simulink model "ESSOneYearInOneMinute_R2015a"  (R2020b)
settings: Solver=ode23tb  StartTime=0  StopTime=365*24*60*60  RelTol=1e-4  EnableMultiTasking=on
StartFcn:
  | tic
StopFcn:
  | toc
values from neighbouring files (symbols this model uses):
  BP1 = [1:24]'    [Build_LoadProfile_Datasets.m]    (also in LoadProfile_Datasets.mat = [1 2 3 4 5 6 7 8 9 10 11 12 ... (24 elements, 24x1)])
  BP2 = [1:3]    [Build_LoadProfile_Datasets.m]    (also in LoadProfile_Datasets.mat = [1 2 3])
  BP3 = [1:2]    [Build_LoadProfile_Datasets.m]    (also in LoadProfile_Datasets.mat = [1 2])
  LoadProfile_Data = [1 2 3 4 5 6 7 8 9 10 11 12 ... (144 elements, 24x3x2)]    [LoadProfile_Datasets.mat]
undefined symbols (not defined in the file or in its folder): A, B, C, D1, Dd, Delta, j, StationData
libraries: powerlib x43, simulink x10, powerlib_meascontrol x8
(part 1 of 2)
settings Model: SimulationMode=accelerator  Creator=at4494  LastModifiedBy=Jared Gooding
settings DataIOCC: LimitDataPoints=on  SaveFormat=Array  SignalLoggingSaveFormat=ModelDataLogs  SaveOutput=off  SaveTime=off  ReturnWorkspaceOutputs=off
settings OptimizationCC: LifeSpan=inf
settings DebuggingCC: UnderspecifiedInitializationDetection=Classic  MergeDetectMultiDrivingBlocksExec=none  SolverPrmCheckMsg=warning  MultiTaskDSMMsg=warning  MultiTaskCondExecSysMsg=none  SFUnexpectedBacktrackingDiag=warning  SFNoUnconditionalDefaultTransitionDiag=warning  SFExecutionAtInitializationDiag=none  ArithmeticOperatorsInVariantConditions=warning
settings HardwareCC: ProdBitPerPointer=32  ProdBitPerSizeT=32  ProdBitPerPtrDiffT=32  ProdLargestAtomicFloat=None  ProdIntDivRoundTo=Undefined  ProdEndianess=Unspecified  ProdWordSize=32  ProdHWDeviceType=32-bit Generic
settings ModelReferenceCC: PropagateSignalLabelsOutOfModel=off
settings SFSimCC: SimUseLocalCustomCode=off  CustomCodeUndefinedFunction=UseInterfaceOnly
settings RTWCC: RTWUseLocalCustomCode=off
settings CodeAppCC: StateflowObjectComments=on
settings GRTTargetCC: TargetLangStandard=C89/C90 (ANSI)
settings ConfigComp: CovMetricSettings=dw  CovSaveCumulativeToWorkspaceVar=on  CovSaveSingleToWorkspaceVar=on  CovExternalEMLEnable=off  CovSFcnEnable=off
settings SimscapeCC: SimscapeNormalizeSystem=off

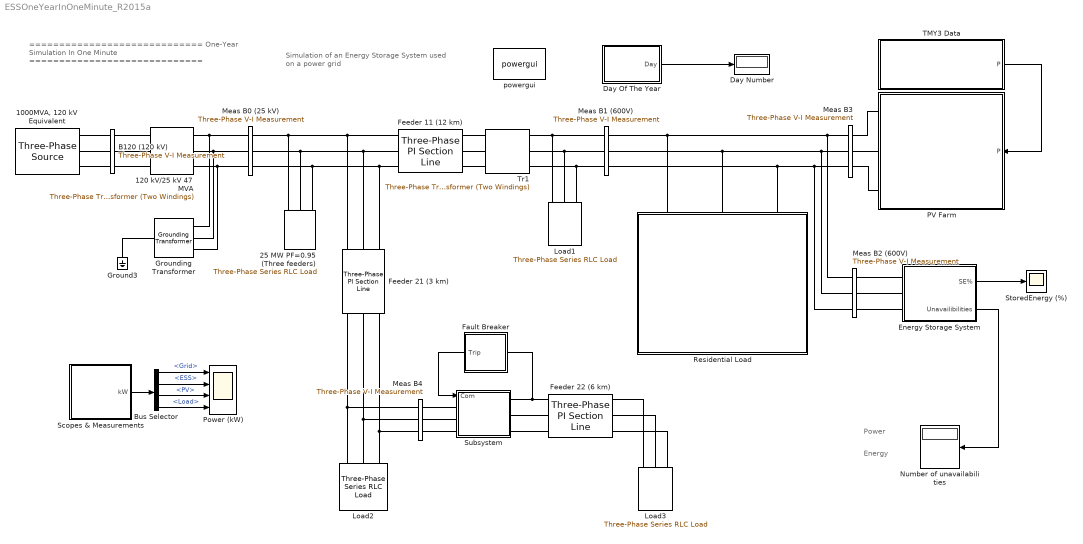
== system ESSOneYearInOneMinute_R2015a ==
  note: Simulation of an Energy Storage
      | System used on a power grid
  note: Power
  note: =============================
      | One-Year Simulation In One Minute
      | =============================
  note: Energy
  " Feeder 11 (12 km)" : powerlib/Elements/Three-Phase PI Section Line  LConnTagsString=a|b|c  RConnTagsString=A|B|C  Length=12  Frequency=60  Resistances=[ 0.104 0.357]  Inductances="[1.048e-3  3.483e-3]"  Capacitances="[ 11.212e-09   4.8118e-09]"
  " Feeder 21 (3 km)" : powerlib/Elements/Three-Phase PI Section Line  LConnTagsString=a|b|c  RConnTagsString=A|B|C  Length=3  Frequency=60  Resistances=[ 0.104 0.357]  Inductances="[1.048e-3  3.483e-3]"  Capacitances="[ 11.212e-09   4.8118e-09]"
  "1000MVA, 120 kV Equivalent" : powerlib/Electrical Sources/Three-Phase Source  InternalConnection=Yg  VoltagePhases=off  Voltage=120e3*1.07  PhaseAngle=0  Voltage_phases=[25e3 25e3 25e3]/sqrt(3)  PhaseAngles_phases=[0 -120 +120]  Frequency=60  NonIdealSource=on  SpecifyImpedance=on  Resistance=0.8929  Inductance=16.58e-3  ShortCircuitLevel=1000e6  BaseVoltage=120e3  XRratio=7  BusType=swing  Pref=0  Qref=0  Prefabc=[10e3, 10e3, 10e3]  Qrefabc=[0, 0, 0]  Qmin=-inf  Qmax=inf
  120 kV/25 kV 47 MVA : powerlib/Elements/Three-Phase Transformer (Two Windings)  Winding1Connection=Yg  Winding2Connection=Delta (D1)  CoreType=Three single-phase transformers  SetSaturation=off  Hysteresis=off  DataFile='basic_model'  SetInitialFlux=off  Measurements=None  UNITS=pu  NominalPower=[47e6 60]  Winding1="[ 120e3  0.185/2/25   0.185/2 ]"  Winding2="[ 25e3  0.185/2/25  0.185/2]"  Rm=500  Lm=500  L0=0.5  Saturation="[ 0,0  ;  0.005,1.2  ;  1.0,1.4 ]"  InitialFluxes=[ 0.8 , -0.8 , 0.7 ]  BreakLoop=off  DiscreteSolver=Trapezoidal iterative  DataType=off  TransfoNumber=0
  25 MW PF=0.95 (Three feeders) : powerlib/Elements/Three-Phase Series RLC Load  LConnTagsString=A|B|C  Configuration=Y (grounded)  NominalVoltage=25e3  Vabc=[1e3 1e3 1e3]  Vabcp=[1e3 1e3 1e3]  NominalFrequency=60  UnbalancedPower=off  ActivePower=25e6  InductivePower=25e6*sqrt(1/0.95^2 - 1)  CapacitivePower=0  Pabc=[10e3 9e3 11e3]  QLabc=[100 90 110]  QCabc=[100 90 110]  Pabcp=[10e3 9e3 11e3]  QLabcp=[100 90 110]  QCabcp=[100 90 110]  Measurements=None  LoadType=constant Z
  B120 (120 kV) : powerlib/Measurements/Three-Phase V-I Measurement  VoltageMeasurement=no  SetLabelV=on  LabelV=Vabc_B120_1  Vpu=on  VpuLL=off  CurrentMeasurement=no  SetLabelI=on  LabelI=Iabc_B120  Ipu=off  Pbase=100e6  Vbase=120e3  OutputType=Complex  PhasorSimulation=on  PSBequivalent=0
  Bus Selector : BusSelector  OutputSignals=Grid,ESS,PV,Load
  Day Number : Display
  Day Of The Year : Subsystem
      mask Display: image(imread('Calendar.ico'))
  Energy Storage System : Subsystem  mask(Generic Energy Storage System){Pnom=275, kWh_Rated=1000, Initial_kWh_pc=90, Efficiency=96, Pmax_Grid=1000, Ki=1000, MinMax=[ 10  90 ], ChargingPower=150}
      mask prompts: Pnom "Rated power in kW"; kWh_Rated "Rated capacity in kWh"; Initial_kWh_pc "Initial stored energy in % of rated capacity"; Efficiency "System efficiency in %"; Pmax_Grid "Maximum power allowed from the grid (kW)"; Ki "Regulator integral gain:"; MinMax "Range of operation [ min  max ] in % of Stored Energy"; ChargingPower "Maximum charging power (kW) during night time:"
      mask help:
      | Model a generic Energy Storage System (ESS) connected to grid through an inverter. The storage technology can be Battery, Flywheel, SuperCapacitor, ...
      |
      | Look Under Mask to see how the model is built.
      mask init:
      | Min=MinMax(1);
      | Max=MinMax(2);
      | Plimit=Pnom*1e3;
      mask DialogControl Container4 Prompt: Power
      mask DialogControl Container7 Prompt: Control
      mask Display: image(imread('Energy.jpg'))
  Fault Breaker : Subsystem  mask(Single-phase Fault Breaker){Day=50, Hour=9, Minute=28, Second=9, FaultDuration=0.2, Ron=0.1}
      mask prompts: FaultDuration "Fault duration (s):"; Ron "Fault resistance (ohm):"
      mask init:
      | T1=(Day-1)*24*60*60;  % Day in seconds
      | T2=(Hour-1)*60*60;    % Hour in seconds
      | T3=(Minute-1)*60;  % Minute in seconds
      | Ton=T1+T2+T3+(Second-1);    % Beginning of fault (s)
      | Toff=Ton+FaultDuration; % End of fault (s)
      mask TypeOptions Day: 1 |      2 |      3 |      4 |      5 |      6 |      7 |      8 |      9 |     10 |     11 |     12 |     13 |     14 |     15 |     16 |     17 |     18 |     19 |     20 |     21 |     22 |     23 |     24 |     25 |     26 |     27 |     28 |     29 |     30 |     31 |     32 |     33 |     34 |     35 |     36 |     37 |     38 |     39 |     40 |     41 |     42 |     43 |     44 |     45 |     46 |     47 |     48 |     49 |     50 |     51 |     52 |     53 |     54 |     55 |     56 |     57 |     58 |     59 |     60 |     61 |     62 |     63 |     64 |     65 |     66 |     67 |     68 |     69 |     70 |     71 |     72 |     73 |     74 |     75 |     76 |     77 |     78 |     79 |     80 |     81 |     82 |     83 |     84 |     85 |     86 |     87 |     88 |     89 |     90 |     91 |     92 |     93 |     94 |     95 |     96 |     97 |     98 |     99 |    100 |    101 |    102 |    103 |    104 |    105 |    106 |    107 |    108 |    109 |    110 |    111 |    112 |    113 |    114 |    115 |    116 |    117 |    118 |    119 |    120 |    121 |    122 |    123 |    124 |    125 |    126 |    127 |    128 |    129 |    130 |    131 |    132 |    133 |    134 |    135 |    136 |    137 |    138 |    139 |    140 |    141 |    142 |    143 |    144 |    145 |    146 |    147 |    148 |    149 |    150 |    151 |    152 |    153 |    154 |    155 |    156 |    157 |    158 |    159 |    160 |    161 |    162 |    163 |    164 |    165 |    166 |    167 |    168 |    169 |    170 |    171 |    172 |    173 |    174 |    175 |    176 |    177 |    178 |    179 |    180 |    181 |    182 |    183 |    184 |    185 |    186 |    187 |    188 |    189 |    190 |    191 |    192 |    193 |    194 |    195 |    196 |    197 |    198 |    199 |    200 |    201 |    202 |    203 |    204 |    205 |    206 |    207 |    208 |    209 |    210 |    211 |    212 |    213 |    214 |    215 |    216 |    217 |    218 |    219 |    220 |    221 |    222 |    223 |    224 |    225 |    226 |    227 |    228 |    229 |    230 |    231 |    232 |    233 |    234 |    235 |    236 |    237 |    238 |    239 |    240 |    241 |    242 |    243 |    244 |    245 |    246 |    247 |    248 |    249 |    250 |    251 |    252 |    253 |    254 |    255 |    256 |    257 |    258 |    259 |    260 |    261 |    262 |    263 |    264 |    265 |    266 |    267 |    268 |    269 |    270 |    271 |    272 |    273 |    274 |    275 |    276 |    277 |    278 |    279 |    280 |    281 |    282 |    283 |    284 |    285 |    286 |    287 |    288 |    289 |    290 |    291 |    292 |    293 |    294 |    295 |    296 |    297 |    298 |    299 |    300 |    301 |    302 |    303 |    304 |    305 |    306 |    307 |    308 |    309 |    310 |    311 |    312 |    313 |    314 |    315 |    316 |    317 |    318 |    319 |    320 |    321 |    322 |    323 |    324 |    325 |    326 |    327 |    328 |    329 |    330 |    331 |    332 |    333 |    334 |    335 |    336 |    337 |    338 |    339 |    340 |    341 |    342 |    343 |    344 |    345 |    346 |    347 |    348 |    349 |    350 |    351 |    352 |    353 |    354 |    355 |    356 |    357 |    358 |    359 |    360 |    361 |    362 |    363 |    364 |    365
      mask TypeOptions Hour: 0 |      1 |      2 |      3 |      4 |      5 |      6 |      7 |      8 |      9 |     10 |     11 |     12 |     13 |     14 |     15 |     16 |     17 |     18 |     19 |     20 |     21 |     22 |     23
      mask TypeOptions Minute: 0 |      1 |      2 |      3 |      4 |      5 |      6 |      7 |      8 |      9 |     10 |     11 |     12 |     13 |     14 |     15 |     16 |     17 |     18 |     19 |     20 |     21 |     22 |     23 |     24 |     25 |     26 |     27 |     28 |     29 |     30 |     31 |     32 |     33 |     34 |     35 |     36 |     37 |     38 |     39 |     40 |     41 |     42 |     43 |     44 |     45 |     46 |     47 |     48 |     49 |     50 |     51 |     52 |     53 |     54 |     55 |     56 |     57 |     58 |     59
      mask TypeOptions Second: 0 |      1 |      2 |      3 |      4 |      5 |      6 |      7 |      8 |      9 |     10 |     11 |     12 |     13 |     14 |     15 |     16 |     17 |     18 |     19 |     20 |     21 |     22 |     23 |     24 |     25 |     26 |     27 |     28 |     29 |     30 |     31 |     32 |     33 |     34 |     35 |     36 |     37 |     38 |     39 |     40 |     41 |     42 |     43 |     44 |     45 |     46 |     47 |     48 |     49 |     50 |     51 |     52 |     53 |     54 |     55 |     56 |     57 |     58 |     59
      mask DialogControl Control2 Prompt: Fault timing:
  Feeder 22 (6 km) : powerlib/Elements/Three-Phase PI Section Line  LConnTagsString=a|b|c  RConnTagsString=A|B|C  Length=6  Frequency=60  Resistances=[ 0.104 0.357]  Inductances="[1.048e-3  3.483e-3]"  Capacitances="[ 11.212e-09   4.8118e-09]"
  Ground3 : powerlib/Elements/Ground  LConnTagsString=a
  "Grounding Transformer " : powerlib/Elements/Grounding Transformer   UNITS=pu  NominalPower="[10e6   60]"  NominalVoltage=25e3  ZeroSequenceImpedance_pu=[0.25 7.5]/(25e3^2/10e6)  MagnetizationBranch_pu=[500 500]  ZeroSequenceImpedance_SI=[0.052083 589.05]  MagnetizationBranch_SI=[1041.7 3.927e+005]  Measurements=None
      settings: SourceProductBaseCode=PS
  Load1 : powerlib/Elements/Three-Phase Series RLC Load  LConnTagsString=A|B|C  Configuration=Y (grounded)  NominalVoltage=600  Vabc=[1e3 1e3 1e3]  Vabcp=[1e3 1e3 1e3]  NominalFrequency=60  UnbalancedPower=off  ActivePower=50e3  InductivePower=0  CapacitivePower=0  Pabc=[10e3 9e3 11e3]  QLabc=[100 90 110]  QCabc=[100 90 110]  Pabcp=[10e3 9e3 11e3]  QLabcp=[100 90 110]  QCabcp=[100 90 110]  Measurements=None  LoadType=constant Z
  Load2 : powerlib/Elements/Three-Phase Series RLC Load  LConnTagsString=A|B|C  Configuration=Y (grounded)  NominalVoltage=25e3  Vabc=[1e3 1e3 1e3]  Vabcp=[1e3 1e3 1e3]  NominalFrequency=60  UnbalancedPower=off  ActivePower=2e6  InductivePower=0.4e6  CapacitivePower=0  Pabc=[10e3 9e3 11e3]  QLabc=[100 90 110]  QCabc=[100 90 110]  Pabcp=[10e3 9e3 11e3]  QLabcp=[100 90 110]  QCabcp=[100 90 110]  Measurements=None  LoadType=constant Z
  Load3 : powerlib/Elements/Three-Phase Series RLC Load  LConnTagsString=A|B|C  Configuration=Y (grounded)  NominalVoltage=25e3  Vabc=[1e3 1e3 1e3]  Vabcp=[1e3 1e3 1e3]  NominalFrequency=60  UnbalancedPower=off  ActivePower=5e6  InductivePower=0.6e6  CapacitivePower=0  Pabc=[10e3 9e3 11e3]  QLabc=[100 90 110]  QCabc=[100 90 110]  Pabcp=[10e3 9e3 11e3]  QLabcp=[100 90 110]  QCabcp=[100 90 110]  Measurements=None  LoadType=constant Z
  "Meas B0 (25 kV) " : powerlib/Measurements/Three-Phase V-I Measurement  VoltageMeasurement=phase-to-ground  SetLabelV=on  LabelV=Vabc_B0  Vpu=off  VpuLL=off  CurrentMeasurement=yes  SetLabelI=on  LabelI=Iabc_B0  Ipu=off  Pbase=10e6  Vbase=25e3  OutputType=Complex  PhasorSimulation=on  PSBequivalent=0
  Meas B1 (600V) : powerlib/Measurements/Three-Phase V-I Measurement  VoltageMeasurement=phase-to-ground  SetLabelV=on  LabelV=Vabc_B1  Vpu=off  VpuLL=off  CurrentMeasurement=yes  SetLabelI=on  LabelI=Iabc_B1  Ipu=off  Pbase=100e6  Vbase=500e3  OutputType=Complex  PhasorSimulation=on  PSBequivalent=0
  Meas B2 (600V) : powerlib/Measurements/Three-Phase V-I Measurement  VoltageMeasurement=phase-to-ground  SetLabelV=on  LabelV=Vabc_B2  Vpu=off  VpuLL=off  CurrentMeasurement=yes  SetLabelI=on  LabelI=Iabc_B2  Ipu=off  Pbase=100e6  Vbase=500e3  OutputType=Complex  PhasorSimulation=on  PSBequivalent=0
  Meas B3 : powerlib/Measurements/Three-Phase V-I Measurement  VoltageMeasurement=phase-to-ground  SetLabelV=on  LabelV=Vabc_B3  Vpu=off  VpuLL=off  CurrentMeasurement=yes  SetLabelI=on  LabelI=Iabc_B3  Ipu=off  Pbase=100e6  Vbase=500e3  OutputType=Complex  PhasorSimulation=on  PSBequivalent=0
  Meas B4 : powerlib/Measurements/Three-Phase V-I Measurement  VoltageMeasurement=phase-to-ground  SetLabelV=on  LabelV=Vabc_B4  Vpu=off  VpuLL=off  CurrentMeasurement=yes  SetLabelI=on  LabelI=Iabc_B4  Ipu=off  Pbase=100e6  Vbase=500e3  OutputType=Complex  PhasorSimulation=on  PSBequivalent=0
  Number of unavailabilities : Display
  PV Farm : Subsystem
      mask Display: image(imread('PV_Farm.jpg'))
  Power (kW) : Scope  NumInputPorts=4
  Residential Load : Subsystem  mask(Dynamic Load based on Load Profiles){DatasetsNumber=Southwest USA, Vnom=600, Pnom_Load=1500, PF=0.95, np_nq=[ 1.8  1.4 ], PlotData_On=off}
      mask prompts: Vnom "Nominal L-L voltage (Vrms)"; Pnom_Load "Nominal load (kVA)"; PF "Power factor ( 0 to 1)"; np_nq "Parameters [ np  nq ]"; PlotData_On "Plot load profile"
      mask help:
      | Implements a three-phase, three-wire dynamic load based on Load Profiles.
      | Active power P and reactive power Q absorbed by the load vary as function of positive-sequence voltage V and load profiles data.
      | The profiles are daily load profiles specified on an hourly basis. For each load profile, the user specifies summer and winter data.
      | P & Q vary as follows:
      | P=P_LoadProfile*(V/Vo)^np
      | Q=Q_LoadProfile*(V/Vo)^nq
      | Note: If np=nq=2, the load behaves as constant impedance load.
      | See documentation below to define additionnal load profiles.
      mask init:
      | BlockName=gcb;
      | load LoadProfile_Datasets
      | np=np_nq(1);
      | nq=np_nq(2);
      | if PlotData_On==1
      |     clf
      |     plot([1:24],LoadProfile_Data(:,2,DatasetsNumber),'r')
      |     hold on
      |     plot([1:24],LoadProfile_Data(:,3,DatasetsNumber),'b')
      |     grid
      |     if DatasetsNumber==1
      |         str='Southwest, USA';
      |     else
      |         str='Northeast, USA';
      |     end
      |     title(['Load profile:',  str ])
      |     ylabel('% of nominal load')
      |     xlabel('Hour of the day')
      |     axis([0 24 0 100])
      |     legend('Summer', 'Winter', 'Location','NorthWest')
      |     set_param(BlockName,'PlotData_On', 'off')
      | end
      settings: AttributesFormatString=Profile:%<DatasetsNumber>
      mask TypeOptions DatasetsNumber: Southwest USA | Northeast USA
      mask DialogControl Control3 Prompt: Documentation
      mask DialogControl Control3 Callback: open('Build_LoadProfile_Datasets.m')
      mask DialogControl Control2 Prompt: Load Profile:
      mask Display: image(imread('Residential.jpg'))
  Scopes & Measurements : Subsystem
  StoredEnergy (%) : Scope
  Subsystem : Subsystem
      mask Display: disp('Three-phase\nBreaker')
  TMY3 Data : Subsystem  mask(TMY3 -to- Power){SortByState=on, ListNum_State=Binghamton Edwin A Link Field, NY, ListNum_Name=Rock Springs Arpt [Green River - UO], WY, IrradianceType=Global Horizontal Irradiance (Wh/m2), TotalArea=3000, Efficiency=20, PlotData_On=off}
      mask prompts: SortByState "Sort site name by state:"; TotalArea "Solar panels total area (m2):"; Efficiency "Overall system efficiency (%):"; PlotData_On "Plot meteorological data"
      mask help:
      | Convert TMY3 solar irradiance data to Power.
      |
      | TMY3 are data files for the typical meteorological year (TMY) data sets
      | derived from the 1961-1990 and 1991-2005 National Solar Radiation
      | Data Base (NSRDB) archives. The files contain hourly values of solar radiation and meteorological elements for a 1-year period.
      |
      | TMY3 files have been produced by NREL's Electric Systems Center under
      | the Solar Resource Characterization Project, which is funded and
      | monitored by the U.S. Department of Energy's Energy Efficiency and
      | Renewable Energy Office.
      |
      | Look Under Mask for additionnal information
      mask init:
      | BlockName=gcb;
      | % Mask parameters visibility:
      | %
      | MV = get_param(BlockName,'MaskVisibilities');
      | MV{3}='off';
      | if SortByState==1
      | 	MV{2}='on';
      |     MV{3}='off';
      |     str_NameState=ListNum_State;
      | else
      |     MV{2}='off';
      |     MV{3}='on';
      |     str_NameState=ListNum_Name;
      | end
      | set_param(BlockName,'MaskVisibilities',MV)
      | %
      | load StationData_NEW
      | max=size(StationData,2);
      | for i=1:max
      |     if strcmp([StationData(i).Name{1}, ', ', StationData(i).State{1}],str_NameState)
      |        Index=StationData(i).NumberByState;
      |     end
      | end
      | if IrradianceType==1
      |     IrradianceTable=StationData(Index).GHIWm2;
      | else
      |     IrradianceTable=StationData(Index).DNIWm2;
      | end
      | if PlotData_On==1
      |     h2=figure;
      |     set(h2,'Name',[StationData(Index).Name{1}, ', ', StationData(Index).State{1}]);
      |     ScreenS=get(0,'Screensize');
      |     set(h2,'Position',[ScreenS(3)/14 ScreenS(4)/12 ScreenS(3)/2.4 ScreenS(4)/1.25])
      |     subplot(3,1,1)
      |     plot([1:size(StationData(Index).GHIWm2,1)]',StationData(Index).GHIWm2)
      |     title('Global Horizontal Irradiance')
      |     ylabel('Wh/m2')
      |     grid
      |     subplot(3,1,2)
      |     plot([1:size(StationData(Index).DHIWm2,1)]',StationData(Index).DHIWm2)
      |     title('Diffuse Horizontal Irradiance')
      |     ylabel('Wh/m2')
      |     grid
      |     subplot(3,1,3)
      |     plot([1:size(StationData(Index).DNIWm2,1)]',StationData(Index).DNIWm2)
      |     title('Direct Normal Irradiance')
      |     ylabel('Wh/m2')
      |     xlabel('Time of the Year in Hours')
      |     %
      |     h3=figure;
      |     set(h3,'Name',[StationData(Index).Name{1}, ', ', StationData(Index).State{1}]);
      |     ScreenS=get(0,'Screensize');
      |     set(h3,'Position',[ScreenS(3)/2 ScreenS(4)/12 ScreenS(3)/2.4 ScreenS(4)/1.25])
      |     subplot(2,1,1)
      |     plot([1:size(StationData(Index).Temperature,1)]',StationData(Index).Temperature)
      |     title('Temperature')
      |     ylabel('C')
      |     grid
      |     subplot(2,1,2)
      |     plot([1:size(StationData(Index).WindSpeed,1)]',StationData(Index).WindSpeed)
      |     title('Wind Speed')
      |     ylabel('m/s')
      |     grid
      |     xlabel('Time of the Year in Hours')
      |     set_param(BlockName,'PlotData_On', 'off')
      | end
      mask TypeOptions ListNum_State: Birmingham Municipal AP, AL | Huntsville Intl/Jones Field, AL | Mobile Regional AP, AL | Montgomery Dannelly Field, AL | Fort Smith Regional AP, AR | Little Rock Adams Field, AR | Phoenix Sky Harbor Intl AP, AZ | Prescott Love Field, AZ | Tucson International AP, AZ | Arcata Airport, CA | Bakersfield Meadows Field, CA | Bishop Airport, CA | Daggett Barstow-Daggett AP, CA | Fresno Yosemite Intl AP, CA | Long Beach Daugherty Fld, CA | Los Angeles Intl Arpt, CA | Redding Municipal Arpt, CA | Sacramento Executive Arpt, CA | San Diego Lindbergh Field, CA | San Francisco Intl AP, CA | Santa Barbara Municipal AP, CA | Santa Maria Public Arpt, CA | Stockton Metropolitan Arpt, CA | Alamosa San Luis Valley Rgnl, CO | Colorado Springs Muni AP, CO | Denver Intl AP, CO | Grand Junction Walker Field, CO | Limon, CO | Pueblo Memorial AP, CO | Bridgeport Sikorsky Memorial, CT | Hartford Bradley Intl AP, CT | Wilmington New Castle Cnty AP, DE | Daytona Beach Intl AP, FL | Fort Myers Page Field, FL | Gainesville Regional AP, FL | Jacksonville Intl Arpt, FL | Key West Intl Arpt, FL | Miami Intl AP, FL | Orlando Intl Arpt, FL | Pensacola Regional AP, FL | Tallahassee Regional AP [ISIS], FL | Tampa International AP, FL | Vero Beach Municipal Arpt, FL | West Palm Beach Intl Arpt, FL | Athens Ben Epps AP, GA | Atlanta Hartsfield Intl AP, GA | Augusta Bush Field, GA | Columbus Metropolitan Arpt, GA | Macon Middle Ga Regional AP, GA | Savannah Intl AP, GA | Hilo International AP, HI | Honolulu Intl Arpt, HI | Kahului Airport, HI | Lihue Airport, HI | Boise Air Terminal [UO], ID | Lewiston Nez Perce Cnty AP, ID | Pocatello Regional AP, ID | Chicago Ohare Intl AP, IL | Moline Quad City Intl AP, IL | Peoria Greater Peoria AP, IL | Rockford Greater Rockford AP, IL | Springfield Capital AP, IL | Evansville Regional AP, IN | Fort Wayne Intl AP, IN | Indianapolis Intl AP, IN | South Bend Michiana Rgnl AP, IN | Des Moines Intl AP, IA | Dubuque Regional AP, IA | Mason City Municipal Arpt, IA | Sioux City Sioux Gateway AP, IA | Waterloo Municipal AP, IA | Concordia Blosser Muni AP, KS | Dodge City Regional AP, KS | Goodland Renner Field, KS | Russell Municipal AP, KS | Topeka Municipal AP, KS | Wichita Mid-Continent AP, KS | Cincinnati Northern Ky AP, KY | Jackson Julian Carroll AP, KY | Lexington Bluegrass AP, KY | Louisville Standiford Field, KY | Paducah Barkley Regional AP, KY | Baton Rouge Ryan Arpt, LA | Lake Charles Regional Arpt, LA | New Orleans Intl Arpt, LA | Shreveport Regional Arpt, LA | Bangor International AP, ME | Caribou Municipal Arpt, ME | Portland Intl Jetport, ME | Baltimore Blt-Washngtn Int'l, MD | Boston Logan Int'l Arpt, MA | Worchester Regional Arpt, MA | Alpena County Regional AP, MI | Detroit City Airport, MI | Detroit Metropolitan Arpt, MI | Flint Bishop Intl Arpt, MI | Grand Rapids Kent County Int', MI | Houghton Lake Roscommon Co Ar, MI | Lansing Capital City Arpt, MI | Muskegon County Arpt, MI | Sault Ste Marie Sanderson Fie, MI | Traverse City Cherry Capital, MI | Duluth International Arpt, MN | International Falls Intl AP, MN | Minneapolis-St Paul Int'l Arp, MN | Rochester International Arpt, MN | St Cloud Regional Arpt, MN | Jackson International AP, MS | Meridian Key Field, MS | Tupelo C D Lemons Arpt, MS | Columbia Regional Airport, MO | Kansas City Int'l Arpt, MO | Springfield Regional Arpt, MO | St Louis Lambert Int'l Arpt, MO | St Louis Spirit of St Louis Airport, MO | Billings Logan Int'l Arpt, MT | Glasgow Intl Arpt, MT | Great Falls Intl Arpt, MT | Havre City-County AP, MT | Helena Regional Airport, MT | Kalispell Glacier Pk Int'l Ar, MT | Missoula International AP, MT | Grand Island Central NE Regio, NE | Lincoln Municipal Arpt, NE | Norfolk Karl Stefan Mem Arpt, NE | North Platte Regional AP, NE | Omaha Eppley Airfield, NE | Scottsbluff W B Heilig Field, NE | Valentine Miller Field, NE | Ely Yelland Field, NV | Las Vegas McCarran Intl AP, NV | Lovelock Derby Field, NV | Mercury Desert Rock AP [SURFRAD], NV | Reno Tahoe International AP, NV | Tonopah Airport, NV | Winnemucca Municipal Arpt, NV | Concord Municipal Arpt, NH | Atlantic City Intl AP, NJ | Newark International Arpt, NJ | Albuquerque Intl Arpt [ISIS], NM | Gallup Sen Clarke Fld, NM | Roswell Industrial Air Park, NM | Albany County AP, NY | Binghamton Edwin A Link Field, NY | Buffalo Niagara Intl AP, NY | Islip Long Isl MacArthur AP, NY | Massena AP, NY | New York J F Kennedy Int'l Ar, NY | New York Laguardia Arpt, NY | Rochester Greater Rochester I, NY | Syracuse Hancock Int'l Arpt, NY | Asheville Regional Arpt, NC | Charlotte Douglas Intl Arpt, NC | Greensboro Piedmont Triad Int, NC | Raleigh Durham International, NC | Wilmington International Arpt, NC | Bismarck Municipal Arpt [ISIS], ND | Fargo Hector International AP, ND | Minot FAA AP, ND | Williston Sloulin Intl AP, ND | Akron Akron-Canton Reg AP, OH | Cleveland Hopkins Intl AP, OH | Columbus Port Columbus Intl A, OH | Dayton International Airport, OH | Mansfield Lahm Municipal Arpt, OH | Toledo Express Airport, OH | Youngstown Regional Airport, OH | Oklahoma City Will Rogers Wor, OK | Tulsa International Airport, OK | Astoria Regional Airport, OR | Burns Municipal Arpt [UO], OR | Eugene Mahlon Sweet Arpt [UO], OR | Medford Rogue Valley Intl AP [Ashland - UO], OR | Pendleton E Or Regional AP, OR | Salem McNary Field, OR | Allentown Lehigh Valley Intl, PA | Bradford Regional AP, PA | Erie International AP, PA | Middletown Harrisburg Intl AP, PA | Philadelphia International AP, PA | Pittsburgh International AP, PA | Wilkes-Barre Scranton Intl AP, PA | Williamsport Regional AP, PA | Providence T F Green State Ar, RI | Charleston Intl Arpt, SC | Columbia Metro Arpt, SC | Greer Greenv'l-Spartanbrg AP, SC | Aberdeen Regional Arpt, SD | Huron Regional Arpt, SD | Pierre Municipal AP, SD | Rapid City Regional Arpt, SD | Sioux Falls Foss Field, SD | Bristol Tri City Airport, TN | Chattanooga Lovell Field AP, TN | Knoxville McGhee Tyson AP, TN | Memphis International AP, TN | Nashville International AP, TN | Abilene Regional AP [UT], TX | Amarillo International AP [Canyon - UT], TX | Austin Mueller Municipal AP [UT], TX | Brownsville S Padre Isl Intl, TX | Corpus Christi Intl Arpt [UT], TX | Dallas-Fort Worth Intl AP, TX | El Paso International AP [UT], TX | Houston Bush Intercontinental, TX | Lubbock International AP, TX | Lufkin Angelina Co, TX | Midland International AP, TX | Port Arthur Jefferson County, TX | San Angelo Mathis Field, TX | San Antonio Intl AP, TX | Victoria Regional AP, TX | Waco Regional AP, TX | Cedar City Municipal AP, UT | Salt Lake City Int'l Arpt [ISIS], UT | Burlington International AP, VT | Lynchburg Regional Arpt, VA | Norfolk International AP, VA | Richmond International AP, VA | Roanoke Regional AP, VA | Washington DC Dulles Int'l Ar [Sterling - ISIS], VA | Washington DC Reagan AP, VA | Olympia Airport, WA | Quillayute State Airport, WA | Seattle Seattle-Tacoma Intl A, WA | Spokane International AP [Cheney - UO], WA | Stampede Pass, WA | Yakima Air Terminal, WA | Beckley Raleigh Co Mem AP, WV | Charleston Yeager Arpt, WV | Elkins Elkins-Randolph Co Arp, WV | Huntington Tri-State Arpt, WV | Eau Claire County AP, WI | Green Bay Austin Straubel Int, WI | La Crosse Municipal Arpt, WI | Madison Dane Co Regional Arpt [ISIS], WI | Milwaukee Mitchell Intl AP, WI | Casper Natrona Co Intl AP, WY | Cheyenne Municipal Arpt, WY | Lander Hunt Field, WY | Rock Springs Arpt [Green River - UO], WY | Sheridan County Arpt, WY
      mask TypeOptions ListNum_Name: Aberdeen Regional Arpt, SD | Abilene Regional AP [UT], TX | Akron Akron-Canton Reg AP, OH | Alamosa San Luis Valley Rgnl, CO | Albany County AP, NY | Albuquerque Intl Arpt [ISIS], NM | Allentown Lehigh Valley Intl, PA | Alpena County Regional AP, MI | Amarillo International AP [Canyon - UT], TX | Arcata Airport, CA | Asheville Regional Arpt, NC | Astoria Regional Airport, OR | Athens Ben Epps AP, GA | Atlanta Hartsfield Intl AP, GA | Atlantic City Intl AP, NJ | Augusta Bush Field, GA | Austin Mueller Municipal AP [UT], TX | Bakersfield Meadows Field, CA | Baltimore Blt-Washngtn Int'l, MD | Bangor International AP, ME | Baton Rouge Ryan Arpt, LA | Beckley Raleigh Co Mem AP, WV | Billings Logan Int'l Arpt, MT | Binghamton Edwin A Link Field, NY | Birmingham Municipal AP, AL | Bishop Airport, CA | Bismarck Municipal Arpt [ISIS], ND | Boise Air Terminal [UO], ID | Boston Logan Int'l Arpt, MA | Bradford Regional AP, PA | Bridgeport Sikorsky Memorial, CT | Bristol Tri City Airport, TN | Brownsville S Padre Isl Intl, TX | Buffalo Niagara Intl AP, NY | Burlington International AP, VT | Burns Municipal Arpt [UO], OR | Caribou Municipal Arpt, ME | Casper Natrona Co Intl AP, WY | Cedar City Municipal AP, UT | Charleston Intl Arpt, SC | Charleston Yeager Arpt, WV | Charlotte Douglas Intl Arpt, NC | Chattanooga Lovell Field AP, TN | Cheyenne Municipal Arpt, WY | Chicago Ohare Intl AP, IL | Cincinnati Northern Ky AP, KY | Cleveland Hopkins Intl AP, OH | Colorado Springs Muni AP, CO | Columbia Metro Arpt, SC | Columbia Regional Airport, MO | Columbus Metropolitan Arpt, GA | Columbus Port Columbus Intl A, OH | Concord Municipal Arpt, NH | Concordia Blosser Muni AP, KS | Corpus Christi Intl Arpt [UT], TX | Daggett Barstow-Daggett AP, CA | Dallas-Fort Worth Intl AP, TX | Dayton International Airport, OH | Daytona Beach Intl AP, FL | Denver Intl AP, CO | Des Moines Intl AP, IA | Detroit City Airport, MI | Detroit Metropolitan Arpt, MI | Dodge City Regional AP, KS | Dubuque Regional AP, IA | Duluth International Arpt, MN | Eau Claire County AP, WI | El Paso International AP [UT], TX | Elkins Elkins-Randolph Co Arp, WV | Ely Yelland Field, NV | Erie International AP, PA | Eugene Mahlon Sweet Arpt [UO], OR | Evansville Regional AP, IN | Fargo Hector International AP, ND | Flint Bishop Intl Arpt, MI | Fort Myers Page Field, FL | Fort Smith Regional AP, AR | Fort Wayne Intl AP, IN | Fresno Yosemite Intl AP, CA | Gainesville Regional AP, FL | Gallup Sen Clarke Fld, NM | Glasgow Intl Arpt, MT | Goodland Renner Field, KS | Grand Island Central NE Regio, NE | Grand Junction Walker Field, CO | Grand Rapids Kent County Int', MI | Great Falls Intl Arpt, MT | Green Bay Austin Straubel Int, WI | Greensboro Piedmont Triad Int, NC | Greer Greenv'l-Spartanbrg AP, SC | Hartford Bradley Intl AP, CT | Havre City-County AP, MT | Helena Regional Airport, MT | Hilo International AP, HI | Honolulu Intl Arpt, HI | Houghton Lake Roscommon Co Ar, MI | Houston Bush Intercontinental, TX | Huntington Tri-State Arpt, WV | Huntsville Intl/Jones Field, AL | Huron Regional Arpt, SD | Indianapolis Intl AP, IN | International Falls Intl AP, MN | Islip Long Isl MacArthur AP, NY | Jackson International AP, MS | Jackson Julian Carroll AP, KY | Jacksonville Intl Arpt, FL | Kahului Airport, HI | Kalispell Glacier Pk Int'l Ar, MT | Kansas City Int'l Arpt, MO | Key West Intl Arpt, FL | Knoxville McGhee Tyson AP, TN | La Crosse Municipal Arpt, WI | Lake Charles Regional Arpt, LA | Lander Hunt Field, WY | Lansing Capital City Arpt, MI | Las Vegas McCarran Intl AP, NV | Lewiston Nez Perce Cnty AP, ID | Lexington Bluegrass AP, KY | Lihue Airport, HI | Limon, CO | Lincoln Municipal Arpt, NE | Little Rock Adams Field, AR | Long Beach Daugherty Fld, CA | Los Angeles Intl Arpt, CA | Louisville Standiford Field, KY | Lovelock Derby Field, NV | Lubbock International AP, TX | Lufkin Angelina Co, TX | Lynchburg Regional Arpt, VA | Macon Middle Ga Regional AP, GA | Madison Dane Co Regional Arpt [ISIS], WI | Mansfield Lahm Municipal Arpt, OH | Mason City Municipal Arpt, IA | Massena AP, NY | Medford Rogue Valley Intl AP [Ashland - UO], OR | Memphis International AP, TN | Mercury Desert Rock AP [SURFRAD], NV | Meridian Key Field, MS | Miami Intl AP, FL | Middletown Harrisburg Intl AP, PA | Midland International AP, TX | Milwaukee Mitchell Intl AP, WI | Minneapolis-St Paul Int'l Arp, MN | Minot FAA AP, ND | Missoula International AP, MT | Mobile Regional AP, AL | Moline Quad City Intl AP, IL | Montgomery Dannelly Field, AL | Muskegon County Arpt, MI | Nashville International AP, TN | New Orleans Intl Arpt, LA | New York J F Kennedy Int'l Ar, NY | New York Laguardia Arpt, NY | Newark International Arpt, NJ | Norfolk International AP, VA | Norfolk Karl Stefan Mem Arpt, NE | North Platte Regional AP, NE | Oklahoma City Will Rogers Wor, OK | Olympia Airport, WA | Omaha Eppley Airfield, NE | Orlando Intl Arpt, FL | Paducah Barkley Regional AP, KY | Pendleton E Or Regional AP, OR | Pensacola Regional AP, FL | Peoria Greater Peoria AP, IL | Philadelphia International AP, PA | Phoenix Sky Harbor Intl AP, AZ | Pierre Municipal AP, SD | Pittsburgh International AP, PA | Pocatello Regional AP, ID | Port Arthur Jefferson County, TX | Portland Intl Jetport, ME | Prescott Love Field, AZ | Providence T F Green State Ar, RI | Pueblo Memorial AP, CO | Quillayute State Airport, WA | Raleigh Durham International, NC | Rapid City Regional Arpt, SD | Redding Municipal Arpt, CA | Reno Tahoe International AP, NV | Richmond International AP, VA | Roanoke Regional AP, VA | Rochester Greater Rochester I, NY | Rochester International Arpt, MN | Rock Springs Arpt [Green River - UO], WY | Rockford Greater Rockford AP, IL | Roswell Industrial Air Park, NM | Russell Municipal AP, KS | Sacramento Executive Arpt, CA | Salem McNary Field, OR | Salt Lake City Int'l Arpt [ISIS], UT | San Angelo Mathis Field, TX | San Antonio Intl AP, TX | San Diego Lindbergh Field, CA | San Francisco Intl AP, CA | Santa Barbara Municipal AP, CA | Santa Maria Public Arpt, CA | Sault Ste Marie Sanderson Fie, MI | Savannah Intl AP, GA | Scottsbluff W B Heilig Field, NE | Seattle Seattle-Tacoma Intl A, WA | Sheridan County Arpt, WY | Shreveport Regional Arpt, LA | Sioux City Sioux Gateway AP, IA | Sioux Falls Foss Field, SD | South Bend Michiana Rgnl AP, IN | Spokane International AP [Cheney - UO], WA | Springfield Capital AP, IL | Springfield Regional Arpt, MO | St Cloud Regional Arpt, MN | St Louis Lambert Int'l Arpt, MO | St Louis Spirit of St Louis Airport, MO | Stampede Pass, WA | Stockton Metropolitan Arpt, CA | Syracuse Hancock Int'l Arpt, NY | Tallahassee Regional AP [ISIS], FL | Tampa International AP, FL | Toledo Express Airport, OH | Tonopah Airport, NV | Topeka Municipal AP, KS | Traverse City Cherry Capital, MI | Tucson International AP, AZ | Tulsa International Airport, OK | Tupelo C D Lemons Arpt, MS | Valentine Miller Field, NE | Vero Beach Municipal Arpt, FL | Victoria Regional AP, TX | Waco Regional AP, TX | Washington DC Dulles Int'l Ar [Sterling - ISIS], VA | Washington DC Reagan AP, VA | Waterloo Municipal AP, IA | West Palm Beach Intl Arpt, FL | Wichita Mid-Continent AP, KS | Wilkes-Barre Scranton Intl AP, PA | Williamsport Regional AP, PA | Williston Sloulin Intl AP, ND | Wilmington International Arpt, NC | Wilmington New Castle Cnty AP, DE | Winnemucca Municipal Arpt, NV | Worchester Regional Arpt, MA | Yakima Air Terminal, WA | Youngstown Regional Airport, OH
      mask TypeOptions IrradianceType: Global Horizontal Irradiance (Wh/m2) | Direct Normal Irradiance (Wh/m2)
      mask DialogControl Control2 Prompt: Site name:
      mask DialogControl Control3 Prompt: Choose irradiance type:
      mask Display: disp([StationData(Index).Name{1},', ',StationData(Index).State{1}])
  Tr1 : powerlib/Elements/Three-Phase Transformer (Two Windings)  Winding1Connection=Yg  Winding2Connection=Yg  CoreType=Three single-phase transformers  SetSaturation=off  Hysteresis=off  DataFile='basic_model'  SetInitialFlux=off  Measurements=None  UNITS=pu  NominalPower=[10e6 60]  Winding1=[ 25e3 0.05/30/2 0.01 ]  Winding2=[ 600 0.05/30/2 0.04 ]  Rm=200  Lm=200  L0=0.5  Saturation="[ 0,0  ;  0.005,1.2  ;  1.0,1.4 ]"  InitialFluxes=[ 0.8 , -0.8 , 0.7 ]  BreakLoop=off  DiscreteSolver=Trapezoidal iterative  DataType=off  TransfoNumber=1
  powergui : powerlib/powergui  Priority=1  SimulationMode=Phasor  SampleTime=50e-6  frequency=60  Iterations=50  frequencyindice=60  Pbase=100e6  ErrMax=1e-4  UnitsV=kV  UnitsW=MW  buscounter=0  FunctionMessages=off  echomessages=off  EnableUseOfTLC=off  CurrentSourceSwitches=off  DisableSnubberDevices=off  DisableRonSwitches=off  DisableVfSwitches=off  DisplayEquations=off  AutomaticDiscreteSolvers=off  SolverType=Tustin  Interpol=off  ExternalGateDelay=off  methode=off  Ts=0  x0status=blocks  SPID=off  SwTol=0  HookPort=off  NonlinearTolerance=1e-4  nMaxIteration=100  ContinueOnMaxIteration=off  RestoreLinks=warning  ResistiveCurrentMeasurement=off  Frange=[0:2:500]  Ylog=off  Xlog=on  ShowGrid=off  save=off  variable=ZData  structure=0  ZoomFFT=off  StartTime=0.0  cycles=1  DisplayStyle=1  fundamental=60  FreqAxis=off  MaxFrequency=1000  frequencyindicesteady=1  RmsSteady=1  display=off
  wires:
  Day Of The Year/1(Day) -> Day Number/1
  Scopes & Measurements/1(kW) -> Bus Selector/1
  Bus Selector/3 -> Power (kW)/3  "<PV>"
  Bus Selector/2 -> Power (kW)/2  "<ESS>"
  Bus Selector/1 -> Power (kW)/1  "<Grid>"
  Bus Selector/4 -> Power (kW)/4  "<Load>"
  TMY3 Data/1(P) -> PV Farm/1(P)
  Energy Storage System/1(SE%) -> StoredEnergy (%)/1
  Fault Breaker/1(Trip) -> Subsystem/1(Com)
  Energy Storage System/2(Unavailibilities) -> Number of unavailabilities/1
  connections:
  Tr1/RConn1 -- Meas B1 (600V)/LConn1 -- Load1/LConn1
  Tr1/RConn2 -- Load1/LConn2 -- Meas B1 (600V)/LConn2
  Tr1/RConn3 -- Load1/LConn3 -- Meas B1 (600V)/LConn3
  " Feeder 11 (12 km)"/RConn1 -- Tr1/LConn1
  " Feeder 11 (12 km)"/RConn2 -- Tr1/LConn2
  " Feeder 11 (12 km)"/RConn3 -- Tr1/LConn3
  "Meas B0 (25 kV) "/RConn1 -- " Feeder 11 (12 km)"/LConn1 -- " Feeder 21 (3 km)"/LConn1 -- 25 MW PF=0.95 (Three feeders)/LConn1
  "Meas B0 (25 kV) "/RConn2 -- " Feeder 21 (3 km)"/LConn2 -- " Feeder 11 (12 km)"/LConn2 -- 25 MW PF=0.95 (Three feeders)/LConn2
  " Feeder 11 (12 km)"/LConn3 -- "Meas B0 (25 kV) "/RConn3 -- 25 MW PF=0.95 (Three feeders)/LConn3 -- " Feeder 21 (3 km)"/LConn3
  Meas B3/RConn1 -- Meas B1 (600V)/RConn1 -- Residential Load/LConn1 -- Meas B2 (600V)/RConn1
  Meas B2 (600V)/RConn3 -- Meas B1 (600V)/RConn3 -- Residential Load/LConn3 -- Meas B3/RConn3
  Meas B2 (600V)/RConn2 -- Meas B1 (600V)/RConn2 -- Residential Load/LConn2 -- Meas B3/RConn2
  Load2/LConn3 -- " Feeder 21 (3 km)"/RConn3 -- Meas B4/LConn3
  " Feeder 21 (3 km)"/RConn1 -- Load2/LConn1 -- Meas B4/LConn1
  " Feeder 21 (3 km)"/RConn2 -- Meas B4/LConn2 -- Load2/LConn2
  Feeder 22 (6 km)/RConn1 -- Load3/LConn1
  Feeder 22 (6 km)/RConn2 -- Load3/LConn2
  Feeder 22 (6 km)/RConn3 -- Load3/LConn3
  120 kV/25 kV 47 MVA/RConn3 -- "Meas B0 (25 kV) "/LConn3 -- "Grounding Transformer "/LConn3
  "Meas B0 (25 kV) "/LConn1 -- "Grounding Transformer "/LConn1 -- 120 kV/25 kV 47 MVA/RConn1
  120 kV/25 kV 47 MVA/RConn2 -- "Meas B0 (25 kV) "/LConn2 -- "Grounding Transformer "/LConn2
  Ground3/LConn1 -- "Grounding Transformer "/RConn1
  "1000MVA, 120 kV Equivalent"/RConn3 -- B120 (120 kV)/LConn3
  120 kV/25 kV 47 MVA/LConn1 -- B120 (120 kV)/RConn1
  120 kV/25 kV 47 MVA/LConn3 -- B120 (120 kV)/RConn3
  120 kV/25 kV 47 MVA/LConn2 -- B120 (120 kV)/RConn2
  "1000MVA, 120 kV Equivalent"/RConn2 -- B120 (120 kV)/LConn2
  "1000MVA, 120 kV Equivalent"/RConn1 -- B120 (120 kV)/LConn1
  PV Farm/RConn1 -- Meas B3/LConn1
  PV Farm/RConn2 -- Meas B3/LConn2
  PV Farm/RConn3 -- Meas B3/LConn3
  Meas B4/RConn1 -- Subsystem/LConn1
  Meas B4/RConn2 -- Subsystem/LConn2
  Meas B4/RConn3 -- Subsystem/LConn3
  Subsystem/RConn1 -- Fault Breaker/LConn1 -- Feeder 22 (6 km)/LConn1
  Subsystem/RConn2 -- Feeder 22 (6 km)/LConn2
  Subsystem/RConn3 -- Feeder 22 (6 km)/LConn3
  Meas B2 (600V)/LConn1 -- Energy Storage System/LConn1
  Meas B2 (600V)/LConn2 -- Energy Storage System/LConn2
  Energy Storage System/LConn3 -- Meas B2 (600V)/LConn3

== system ESSOneYearInOneMinute_R2015a/Day Of The Year ==
  Add : Sum
  Compare To Zero : simulink/Logic and Bit Operations/Compare To Zero  relop===  OutDataTypeStr=boolean
  Constant : Constant
  Counter : Subsystem
  Hour -to- Day : Gain  Gain=1/24
  Rounding Function : Rounding  Operator=fix
  Sawtooth Generator : powerlib_meascontrol/Pulse & Signal Generators/Sawtooth Generator  Freq=1/60/60  Phase=180  Ts=0
  Day : Outport
  wires:
  Sawtooth Generator/1 -> Add/1
  Compare To Zero/1 -> Counter/Enable
  Add/1 -> Compare To Zero/1
  Constant/1 -> Add/2
  Counter/1(Out1) -> Hour -to- Day/1
  Hour -to- Day/1 -> Rounding Function/1
  Rounding Function/1 -> Day/1

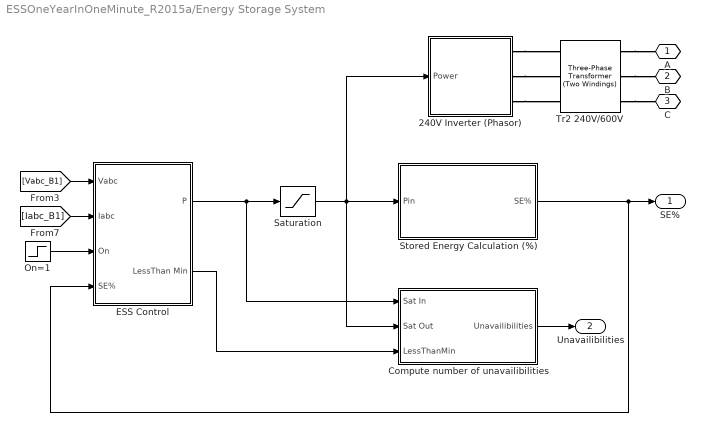
== system ESSOneYearInOneMinute_R2015a/Energy Storage System ==
  240V Inverter (Phasor) : Subsystem
  Compute number of unavailibilities : Subsystem
  ESS Control : Subsystem
  On=1 : Step  Time=0.01*24*60*60  Before=1  SampleTime=0
  Saturation : Saturate  UpperLimit=Pnom*1e3  LowerLimit=-Pnom*1e3
  Stored Energy Calculation (%) : Subsystem
  Tr2 240V/600V : powerlib/Elements/Three-Phase Transformer (Two Windings)  Winding1Connection=Yg  Winding2Connection=Yg  CoreType=Three single-phase transformers  SetSaturation=off  Hysteresis=off  DataFile='basic_model'  SetInitialFlux=off  Measurements=None  UNITS=pu  NominalPower=[Pnom*1e3 60]  Winding1=[ 600 0.05/30/2 0.01 ]  Winding2=[ 240 0.05/30/2 0.04 ]  Rm=100  Lm=100  L0=0.5  Saturation="[ 0,0  ;  0.005,1.2  ;  1.0,1.4 ]"  InitialFluxes=[ 0.8 , -0.8 , 0.7 ]  BreakLoop=off  DiscreteSolver=Trapezoidal iterative  DataType=off  TransfoNumber=1
  A : PMIOPort  Tag=PMCPort  Side=Left
  B : PMIOPort  Tag=PMCPort  Port=2  Side=Left
  C : PMIOPort  Tag=PMCPort  Port=3  Side=Left
  SE% : Outport
  Unavailibilities : Outport  Port=2
  wires:
  Saturation/1 -> Stored Energy Calculation (%)/1(Pin), 240V Inverter (Phasor)/1(Power), Compute number of unavailibilities/2(Sat Out)
  ESS Control/1(P) -> Saturation/1, Compute number of unavailibilities/1(Sat In)
  [Vabc_B1] -> ESS Control/1(Vabc)
  [Iabc_B1] -> ESS Control/2(Iabc)
  On=1/1 -> ESS Control/3(On)
  ESS Control/2(LessThan Min) -> Compute number of unavailibilities/3(LessThanMin)
  Compute number of unavailibilities/1(Unavailibilities) -> Unavailibilities/1
  Stored Energy Calculation (%)/1(SE%) -> SE%/1, ESS Control/4(SE%)
  connections:
  240V Inverter (Phasor)/RConn1 -- Tr2 240V/600V/RConn1
  240V Inverter (Phasor)/RConn2 -- Tr2 240V/600V/RConn2
  240V Inverter (Phasor)/RConn3 -- Tr2 240V/600V/RConn3
  Tr2 240V/600V/LConn1 -- A/RConn1
  Tr2 240V/600V/LConn2 -- B/RConn1
  Tr2 240V/600V/LConn3 -- C/RConn1

== system ESSOneYearInOneMinute_R2015a/Fault Breaker ==
  Clock : Clock
  Compare To Constant : simulink/Logic and Bit Operations/Compare To Constant  relop=>=  const=Ton  OutDataTypeStr=boolean
  Compare To Constant1 : simulink/Logic and Bit Operations/Compare To Constant  relop=<  const=Toff  OutDataTypeStr=boolean
  Fault Breaker : powerlib/Elements/Breaker  InitialState=0  SwitchingTimes=[0 0.2]+ 8760*60*60/2  External=on  BreakerResistance=Ron  SnubberResistance=1e6  SnubberCapacitance=inf  Measurements=None  MoreParameters=off  NoBreakLoop=off
  Ground : powerlib/Elements/Ground  LConnTagsString=a
  Logical Operator : Logic  AllPortsSameDT=off  OutDataTypeStr=float('double')
  A : PMIOPort  Side=Left
  Trip : Outport
  wires:
  Logical Operator/1 -> Fault Breaker/1
  Compare To Constant/1 -> Logical Operator/1
  Clock/1 -> Compare To Constant1/1, Compare To Constant/1
  Compare To Constant1/1 -> Trip/1, Logical Operator/2
  connections:
  Fault Breaker/LConn1 -- A/RConn1
  Ground/LConn1 -- Fault Breaker/RConn1

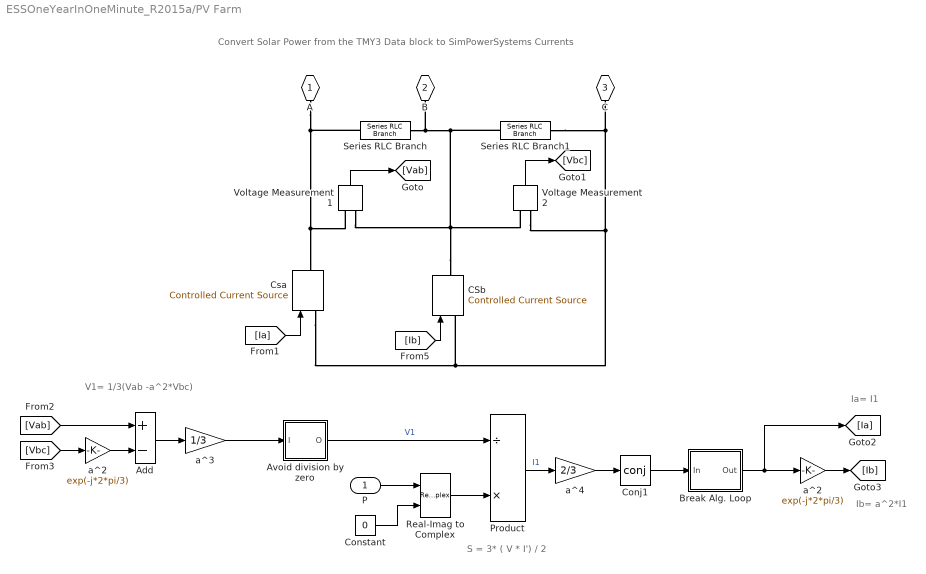
== system ESSOneYearInOneMinute_R2015a/PV Farm ==
  note: Ib= a^2*I1
  note: Ia= I1
  note: S = 3* ( V * I') / 2
  note: V1= 1/3(Vab -a^2*Vbc)
  note: Convert Solar Power from the TMY3 Data block to SimPowerSystems Currents
  P : Inport
  Add : Sum  Inputs=+-
  Avoid division by zero : Subsystem
  "Break Alg. Loop " : Subsystem
  CSb : powerlib/Electrical Sources/Controlled Current Source  Initialize=off  Source_Type=AC  Amplitude=0  Phase=0  Frequency=0  Measurements=None
  Conj1 : Math  Operator=conj  SignedPower=on  SaturateOnIntegerOverflow=on
  Constant : Constant  Value=0
  Csa : powerlib/Electrical Sources/Controlled Current Source  Initialize=off  Source_Type=AC  Amplitude=0  Phase=0  Frequency=0  Measurements=None
  Product : Product  Inputs=/*  InputSameDT=on  SaturateOnIntegerOverflow=on  OutDataTypeStr=Inherit: Same as first input
  Real-Imag to Complex : RealImagToComplex
  Series RLC Branch : powerlib/Elements/Series RLC Branch  LConnTagsString=__new0  RConnTagsString=__new0  BranchType=R  Resistance=1e6  Inductance=1e-3  SetiL0=off  InitialCurrent=0  Capacitance=1e-6  Setx0=off  InitialVoltage=0  Measurements=None
  Series RLC Branch1 : powerlib/Elements/Series RLC Branch  LConnTagsString=__new0  RConnTagsString=__new0  BranchType=R  Resistance=1e6  Inductance=1e-3  SetiL0=off  InitialCurrent=0  Capacitance=1e-6  Setx0=off  InitialVoltage=0  Measurements=None
  Voltage Measurement1 : powerlib/Measurements/Voltage Measurement  PhasorSimulation=on  OutputType=Complex  PSBequivalent=0
  Voltage Measurement2 : powerlib/Measurements/Voltage Measurement  PhasorSimulation=on  OutputType=Complex  PSBequivalent=0
  a^2 : Gain  Gain=exp(-j*2*pi/3)  SaturateOnIntegerOverflow=on  OutDataTypeStr=Inherit: Same as input  ParamDataTypeStr=Inherit: Same as input
  "a^2 " : Gain  Gain=exp(-j*2*pi/3)  SaturateOnIntegerOverflow=on  OutDataTypeStr=Inherit: Same as input  ParamDataTypeStr=Inherit: Same as input
  a^3 : Gain  Gain=1/3  SaturateOnIntegerOverflow=on  OutDataTypeStr=Inherit: Same as input  ParamDataTypeStr=Inherit: Same as input
  a^4 : Gain  Gain=2/3  SaturateOnIntegerOverflow=on  OutDataTypeStr=Inherit: Same as input  ParamDataTypeStr=Inherit: Same as input
  A : PMIOPort  Tag=PMCPort  Side=Right
  B : PMIOPort  Tag=PMCPort  Port=2  Side=Right
  C : PMIOPort  Tag=PMCPort  Port=3  Side=Right
  wires:
  [Ib] -> CSb/1
  "Break Alg. Loop "/1(Out) -> a^2/1, [Ia]
  a^4/1 -> Conj1/1
  "a^2 "/1 -> Add/2
  [Vbc] -> "a^2 "/1
  [Vab] -> Add/1
  Add/1 -> a^3/1
  a^3/1 -> Avoid division by zero/1(I)
  Conj1/1 -> "Break Alg. Loop "/1(In)
  Avoid division by zero/1(O) -> Product/1  "V1"
  a^2/1 -> [Ib]
  [Ia] -> Csa/1
  Product/1 -> a^4/1  "I1"
  Real-Imag to Complex/1 -> Product/2
  Voltage Measurement2/1 -> [Vbc]
  Voltage Measurement1/1 -> [Vab]
  P/1 -> Real-Imag to Complex/1
  Constant/1 -> Real-Imag to Complex/2
  connections:
  CSb/RConn1 -- Voltage Measurement1/LConn2 -- Voltage Measurement2/LConn1 -- Series RLC Branch/RConn1 -- B/RConn1 -- Series RLC Branch1/LConn1
  Voltage Measurement2/LConn2 -- Csa/LConn1 -- CSb/LConn1 -- C/RConn1 -- Series RLC Branch1/RConn1
  A/RConn1 -- Series RLC Branch/LConn1 -- Voltage Measurement1/LConn1 -- Csa/RConn1

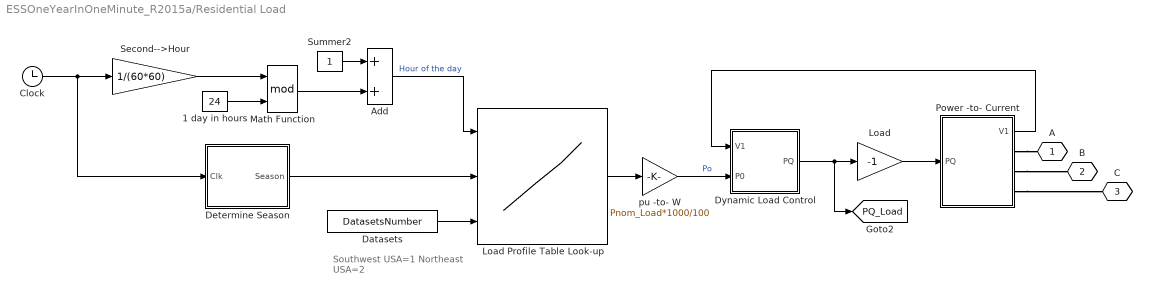
== system ESSOneYearInOneMinute_R2015a/Residential Load ==
  note: Southwest USA=1
      | Northeast USA=2
  1 day in hours : Constant  Value=24
  Add : Sum
  Clock : Clock
  Datasets : Constant  Value=DatasetsNumber
  Determine Season : Subsystem
  Dynamic Load Control : Subsystem
  Load : Gain  Gain=-1
  Load Profile Table Look-up : Lookup_n-D  NumberOfTableDimensions=3  BreakpointsForDimension1=BP1  BreakpointsForDimension2=BP2  BreakpointsForDimension3=BP3  Table=LoadProfile_Data  InternalRulePriority=Speed  RndMeth=Simplest  InputSameDT=on
      settings: InputPortMap=u0,u1,u2
  Math Function : Math  Operator=mod  SignedPower=on  SaturateOnIntegerOverflow=on
  Power -to- Current : Subsystem
  Second-->Hour : Gain  Gain=1/(60*60)
  Summer2 : Constant
  pu -to- W : Gain  Gain=Pnom_Load*1000/100
  A : PMIOPort  Tag=PMCPort  Side=Left
  B : PMIOPort  Tag=PMCPort  Port=2  Side=Left
  C : PMIOPort  Tag=PMCPort  Port=3  Side=Left
  tag scope: PQ_Load=global
  wires:
  1 day in hours/1 -> Math Function/2
  Load Profile Table Look-up/1 -> pu -to- W/1
  Datasets/1 -> Load Profile Table Look-up/3
  Clock/1 -> Determine Season/1(Clk), Second-->Hour/1
  Load/1 -> Power -to- Current/1(PQ)
  Second-->Hour/1 -> Math Function/1
  Math Function/1 -> Add/2
  Add/1 -> Load Profile Table Look-up/1  "Hour of the day"
  Summer2/1 -> Add/1
  Determine Season/1(Season) -> Load Profile Table Look-up/2
  Dynamic Load Control/1(PQ) -> [PQ_Load], Load/1
  Power -to- Current/1(V1) -> Dynamic Load Control/1(V1)
  pu -to- W/1 -> Dynamic Load Control/2(P0)  "Po"
  connections:
  Power -to- Current/RConn1 -- A/RConn1
  Power -to- Current/RConn2 -- B/RConn1
  Power -to- Current/RConn3 -- C/RConn1
